simulink library "SilExtended_libbrowser"  (R2022b)
settings: Solver=VariableStepAuto  StartTime=0.0  StopTime=10.0  RelTol=1e-3
settings Model: Creator=BEATOA  LastModifiedBy=FAGNAL

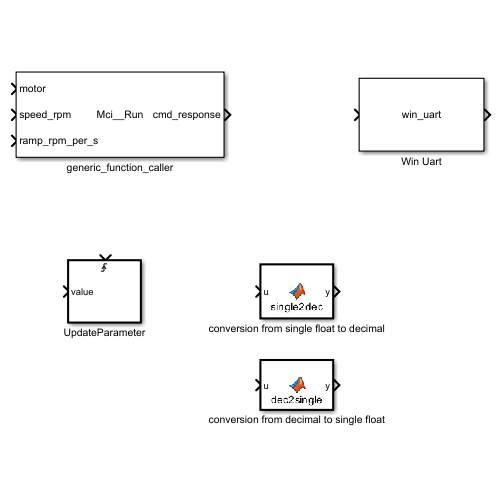
[thumbnail: Simulink's stored preview of the top-level diagram]
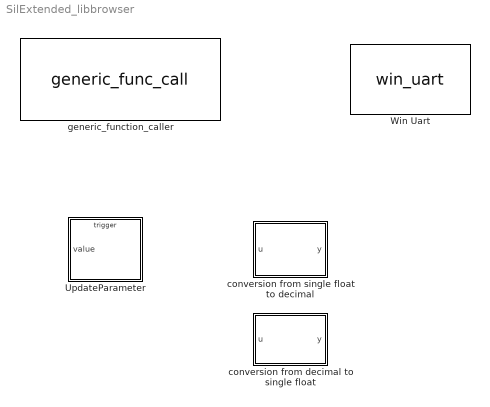
== system SilExtended_libbrowser ==
  UpdateParameter : Subsystem  mask{TunePrm=''}
      mask prompts: TunePrm "Parameter Name"
      settings: CopyFcn=set_param(gcbh,'LinkStatus','none');
  Win Uart : S-Function  FunctionName=win_uart  SFunctionDeploymentMode=off  EnableBusSupport=off
  conversion from decimal to single float : MATLAB Function  TreatAsAtomicUnit=on
  conversion from single float to decimal : MATLAB Function  TreatAsAtomicUnit=on
  generic_function_caller : S-Function  FunctionName=generic_func_call  Parameters=0 ,3 ,1  SFunctionDeploymentMode=off  EnableBusSupport=off  mask{func_list=Mci__Run}
      mask init:
      | func_names = evalin('base', 'generic_func_array(:,1)');
      |     maskObj = Simulink.Mask.get(gcb);
      |     maskObj.Parameters.TypeOptions = func_names;
      settings: CopyFcn=set_param(gcb, 'LinkStatus','none')
      mask TypeOptions func_list: Mci__Run | Mci__Stop | Mci__GetDigital | Mci__GetAnalog | Mci__SetDigital | Mci__SetAnalog | Mci__FvtStart | Reserved1 | CommandManager__RunLoad | Reserved2
      mask Callback func_list:
      | func_array = evalin('base', 'generic_func_array');
      |     maskObj = Simulink.Mask.get(gcb);
      |     selected_idx = find(strcmp(maskObj.Parameters.Value,maskObj.Parameters.TypeOptions));
      | 
      |     % preparing to inject s-function parameters
      |     idx = selected_idx-1;
      |     NAME_POS = 1;
      |     IN_POS = 2;
      |     OUT_POS = 3;
      |     in_names = func_array{selected_idx, IN_POS};
      |     in_size = length(in_names);
      |     out_names = func_array{selected_idx, OUT_POS};
      |     out_size = length(out_names);
      |     % injecting s-function parameter
      |     set_param(gcb,'Parameters',[int2str(idx) ' ,' int2str(in_size) ' ,' int2str(out_size)]);
      | 
      |     maskdispl =['disp(''''' func_array{selected_idx, NAME_POS} ''''');'];
      |     % updating block name accordingly
      | 
      | 
      |     % updating port labels accordingly
      |     for i=1:length(in_names)
      |         maskdispl = [maskdispl 'port_label(''''input'''',' int2str(i) ',''''' in_names{i} ''''');'];
      |     end
      |     for i=1:length(out_names)
      |         maskdispl = [maskdispl 'port_label(''''output'''',' int2str(i) ',''''' out_names{i} ''''');'];
      |     end
      |     complete_str = ['set_param(gcbh,''MaskDisplay'',[''' maskdispl ''']);'];
      | 
      |     evalin('caller', complete_str);
      mask Display: disp('Mci__Run');port_label('input',1,'motor');port_label('input',2,'speed_rpm');port_label('input',3,'ramp_rpm_per_s');port_label('output',1,'cmd_response');

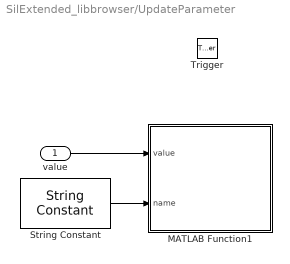
== system SilExtended_libbrowser/UpdateParameter ==
  value : Inport
  Trigger : TriggerPort  VariantControl=(inherit)  PortDimensions=1
  MATLAB Function1 : MATLAB Function  TreatAsAtomicUnit=on
  String Constant : StringConstant  String=TunePrm
  wires:
  value/1 -> MATLAB Function1/1(value)
  String Constant/1 -> MATLAB Function1/2(name)

== matlab function SilExtended_libbrowser/conversion from single float to decimal ==
  data: u input; y output size=1
function y = single2dec(u)


y =double(typecast(single(u),'int32'));

== matlab function SilExtended_libbrowser/conversion from decimal to single float ==
  data: u input; y output size=1
function y = dec2single(u)


y =typecast(uint32(u),'single');

== matlab function SilExtended_libbrowser/UpdateParameter/MATLAB Function1 ==
  data: value input; name input string
function fcn(value,name)
% updatePrm m function is located in tools\CustomMFunctions and it must be
% added to the path before calling it
coder.extrinsic('updatePrm');
coder.extrinsic('set_param');

updatePrm(value,name);
set_param(bdroot, 'SimulationCommand', 'update');
